simulink model "lab3_ss_nominal_box_sim"  (R2024b)
settings: Solver=ode45  StartTime=0.0  StopTime=20  RelTol=1e-3
undefined symbols (not defined in the file): degs2rpm, deltaSS, DiscIntNeverNeededParam, nominal_K, nominal_Nu, nominal_Nx, rpm2rads, sens, step_amplitude, t0_value, t1_value, Ts, wcSS
libraries: simulink x1
settings Model: Creator=andre  LastModifiedBy=andre

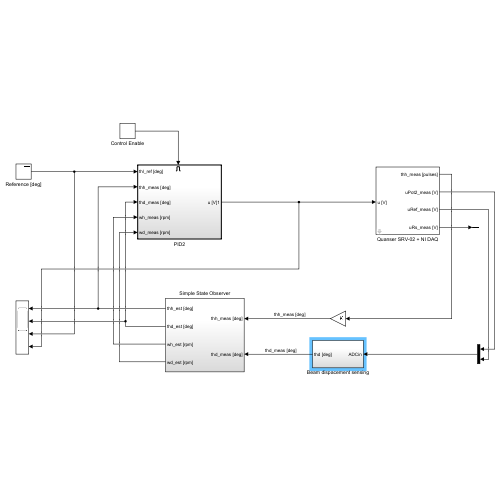
[thumbnail: Simulink's stored preview of the top-level diagram]
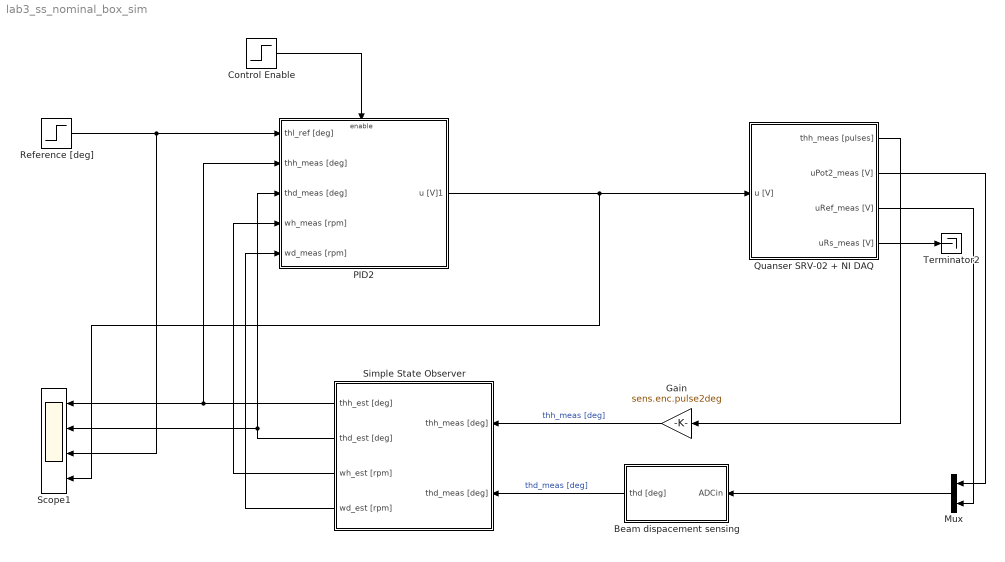
== system lab3_ss_nominal_box_sim ==
  Beam dispacement sensing : Subsystem
  Control Enable : Step  Time=0.7  SampleTime=0
  Gain : Gain  Gain=sens.enc.pulse2deg
  Mux : Mux  Inputs=2
  PID2 : Subsystem
  Quanser SRV-02 + NI DAQ : Subsystem  mask(Quanser SRV-02 (with resonant load) + NI DAQ){Ts=Ts, fricType=Karnopp, lockShaft=off, beamInitPos=10}
      mask prompts: Ts "NI DAQ Sample Time:"; fricType "Friction model"; lockShaft "Lock motor shaft"; beamInitPos "Beam initial position [deg]:"
      mask help: Quanser SRV-02 (with resonant load) + NI DAQ model.
      mask init:
      | %%
      | % Riccardo Antonello (riccardo.antonello@unipd.it)
      | %
      | % April 28, 2020
      | %
      | % Dept. of Information Engineering, University of Padova
      | %
      | 
      | %%  Conversion gains
      | deg2rad = pi/180;                   %   [deg]   -> [rad]
      | rad2deg = 180/pi;                   %   [rad]   -> [deg]
      | 
      | 
      | %%  Sensors data
      | 
      | %   shunt resistor
      | sens.curr.Rs = 0.5;   
      | 
      | %   Hewlett-Packard HEDS-5540#A06 optical encoder
      | sens.enc.ppr = 500*4;                                                   %   pulses per rotation
      | sens.enc.pulse2deg = 360/sens.enc.ppr;                                  %   [pulses] -> [deg]
      | sens.enc.pulse2rad = 2*pi/sens.enc.ppr;                                 %   [pulses] -> [rad]
      | sens.enc.deg2pulse = sens.enc.ppr/360;                                  %   [deg] -> [pulses]
      | sens.enc.rad2pulse = sens.enc.ppr/2/pi;                                 %   [rad] -> [pulses]
      | 
      | %   potentiometer 2 (Spectrol 357-0-0-103) - installed on hub
      | sens.pot2.range.R      = 10e3;                                          %   ohmic value range 
      | sens.pot2.range.V      = 5;                                             %   voltage range
      | sens.pot2.range.th_deg = 340;                                           %   angle range [deg]
      | sens.pot2.range.th     = sens.pot2.range.th_deg * deg2rad;              %   angle range [rad]                           
      | sens.pot2.deg2V        = sens.pot2.range.V / sens.pot2.range.th_deg;    %   sensitivity [V/deg]
      | sens.pot2.rad2V        = sens.pot2.range.V / sens.pot2.range.th;        %   sensitivity [V/rad]
      | sens.pot2.V2deg        = 1/sens.pot2.deg2V;                             %   conversion gain [V] -> [deg]
      | sens.pot2.V2rad        = 1/sens.pot2.rad2V;                             %   conversion gain [V] -> [rad]
      | sens.pot2.noise.var    = 3.5e-7;                                        %   out noise variance [V^2]
      | 
      | 
      | %%  Data acquisition board (daq) data
      | 
      | %   NI PCI-6221 DAC data
      | daq.dac.bits = 16;                                  %   resolution (bits)
      | daq.dac.fs   = 10;                                  %   full scale 
      | daq.dac.q    = 2*daq.dac.fs/(2^daq.dac.bits-1);     %	quantization
      | 
      | %   NI PCI-6221 ADC data
      | daq.adc.bits = 16;                                  %   resolution (bits)
      | daq.adc.fs   = 10;                                  %   full scale (as set in SLDRT Analog Input block)
      | daq.adc.q    = 2*daq.adc.fs/(2^daq.adc.bits-1);     %   quantization   
      | 
      | 
      | %%  Set beam initial position
      | % SRV02Handle = find_system(gcb, ...
      | %     'LookUnderMasks', 'on', ...
      | %     'FindAll', 'on', ...
      | %     'FollowLinks', 'on', ...
      | %     'SearchDepth', '1', ...
      | %     'BlockType', 'ModelReference', ...
      | %     'Name', 'Quanser SRV-02');
      | %
      | % %get_param(SRV02Handle, 'InstanceParameters')
      | % InstanceParams = get_param(SRV02Handle, 'InstanceParameters');
      | % for k = 1:length(InstanceParams)
      | %     if strcmp(InstanceParams(k).Name, 'thb0')
      | %         if lockShaft
      | %             InstanceParams(k).Value = sprintf('%f', beamInitPos);
      | %         else
      | %             InstanceParams(k).Value = sprintf('%f', 0);    
      | %         end
      | %         set_param(SRV02Handle, 'InstanceParameters', InstanceParams);
      | %         break;
      | %     end
      | % end
      | 
      | if lockShaft
      |     thb0 = beamInitPos;
      | else
      |     thb0 = 0;    
      | end
      | 
      | 
      | %%  Mask initialization
      | if lockShaft
      |     
      |     %   find Inport handle
      |     InPortHandle = find_system(gcb, ...
      |         'LookUnderMasks', 'on', ...
      |         'FindAll', 'on', ...
      |         'FollowLinks', 'on', ...
      |         'SearchDepth', '1', ...
      |         'BlockType', 'Inport', ...
      |         'Name', 'u [V]');
      |     
      |     if ~isempty(InPortHandle)
      |     
      |         %   find DAC handle
      |         DACHandle = find_system(gcb, ...
      |             'LookUnderMasks', 'on', ...
      |             'FindAll', 'on', ...
      |             'FollowLinks', 'on', ...
      |             'SearchDepth', '1', ...
      |             'BlockType', 'SubSystem', ...
      |             'Name', 'DAC');  
      | 
      |         %   remove Inport output connection   
      |         InportConn = get_param(InPortHandle, 'PortConnectivity');
      |         delete_line(gcb, InportConn.Position);
      | 
      |         %   remove Inport block
      |         delete_block(InPortHandle);
      | 
      |         %   add Constant block
      |         ConstantHandle = add_block( ...
      |             'simulink/Sources/Constant', [gcb, '/u [V]'], ...
      |             'Position', [20   -37    50   -23], ...
      |             'Value', '0');
      | 
      |         %   connect Constant to DAC block
      |         DACPortHandles = get_param(DACHandle, 'PortHandles');
      |         ConstantPortHandles = get_param(ConstantHandle, 'PortHandles');
      |         add_line(gcb, ConstantPortHandles.Outport(1), DACPortHandles.Inport(1));
      |     
      |     end
      |     
      | else
      |     
      |     %   find Constant handle
      |     ConstantHandle = find_system(gcb, ...
      |         'LookUnderMasks', 'on', ...
      |         'FindAll', 'on', ...
      |         'FollowLinks', 'on', ...
      |         'SearchDepth', '1', ...
      |         'BlockType', 'Constant', ...
      |         'Name', 'u [V]');
      |     
      |     if ~isempty(ConstantHandle)
      |     
      |         %   find DAC handle
      |         DACHandle = find_system(gcb, ...
      |             'LookUnderMasks', 'on', ...
      |             'FindAll', 'on', ...
      |             'FollowLinks', 'on', ...
      |             'SearchDepth', '1', ...
      |             'BlockType', 'SubSystem', ...
      |             'Name', 'DAC');  
      |  
      |         %   remove Constant output connection   
      |         ConstantConn = get_param(ConstantHandle, 'PortConnectivity');
      |         delete_line(gcb, ConstantConn.Position);
      | 
      |         %   remove Inport block
      |         delete_block(ConstantHandle);   
      | 
      |         %   add Inport block
      |         InportHandle = add_block( ...
      |             'simulink/Sources/In1', [gcb, '/u [V]'], ...
      |             'Position', [20   -37    50   -23], ...
      |             'Port', '1');
      | 
      |         %   connect Constant to DAC block
      |         DACPortHandles = get_param(DACHandle, 'PortHandles');
      |         InportPortHandles = get_param(InportHandle, 'PortHandles');
      |         add_line(gcb, InportPortHandles.Outport(1), DACPortHandles.Inport(1));
      |     
      |      end
      |     
      | end
      mask Help:
      | Riccardo Antonello (antonello@dei.unipd.it)
      | 
      | April 28, 2020
      | 
      | Dept. of Information Engineering, University of Padova
      mask TypeOptions fricType: Coulomb + viscous | Karnopp
      mask Callback lockShaft:
      | %   get status of check box
      | lockShaft = get_param(gcb, 'lockShaft');
      | 
      | %   get current value of MaskVisibilities property
      | maskVisibilities = get_param(gcb, 'MaskVisibilities');
      | 
      | %   set visibility of the dialog box element
      | if strcmp(lockShaft, 'on')
      |     maskVisibilities{4} = 'on';
      | else
      |     maskVisibilities{4} = 'off';
      | end
      | 
      | % Set the 'MaskVisibilities' property for each parameter in mask
      | set_param( gcb, 'MaskVisibilities', maskVisibilities);
  Reference [deg] : Step  Time=0  After=step_amplitude  SampleTime=Ts
  Scope1 : Scope  NumInputPorts=4
  Simple State Observer : Subsystem
  Terminator2 : Terminator
  wires:
  Gain/1 -> Simple State Observer/1(thh_meas [deg])  "thh_meas [deg]"
  Reference [deg]/1 -> Scope1/3, PID2/1(thl_ref [deg])
  Quanser SRV-02 + NI DAQ/1(thh_meas [pulses]) -> Gain/1
  Mux/1 -> Beam dispacement sensing/1(ADCin)
  Quanser SRV-02 + NI DAQ/4(uRs_meas [V]) -> Terminator2/1
  Quanser SRV-02 + NI DAQ/3(uRef_meas [V]) -> Mux/2
  Simple State Observer/1(thh_est [deg]) -> PID2/2(thh_meas [deg]), Scope1/1
  Control Enable/1 -> PID2/Enable
  Quanser SRV-02 + NI DAQ/2(uPot2_meas [V]) -> Mux/1
  Beam dispacement sensing/1(thd [deg]) -> Simple State Observer/2(thd_meas [deg])  "thd_meas [deg]"
  PID2/1(u [V]1) -> Quanser SRV-02 + NI DAQ/1(u [V]), Scope1/4
  Simple State Observer/2(thd_est [deg]) -> Scope1/2, PID2/3(thd_meas [deg])
  Simple State Observer/3(wh_est [rpm]) -> PID2/4(wh_meas [rpm])
  Simple State Observer/4(wd_est [rpm]) -> PID2/5(wd_meas [rpm])

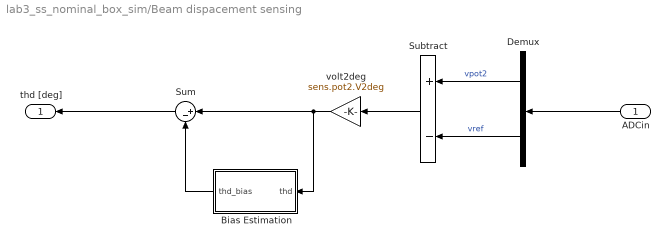
== system lab3_ss_nominal_box_sim/Beam dispacement sensing ==
  ADCin : Inport
  Bias Estimation : Subsystem
  Demux : Demux  Outputs=2
  Subtract : Sum  Inputs=+-
  Sum : Sum  Inputs=|+-
  volt2deg : Gain  Gain=sens.pot2.V2deg
  thd [deg] : Outport
  wires:
  Subtract/1 -> volt2deg/1
  volt2deg/1 -> Sum/1, Bias Estimation/1(thd)
  Sum/1 -> thd [deg]/1
  Bias Estimation/1(thd_bias) -> Sum/2
  ADCin/1 -> Demux/1
  Demux/1 -> Subtract/1  "vpot2"
  Demux/2 -> Subtract/2  "vref"

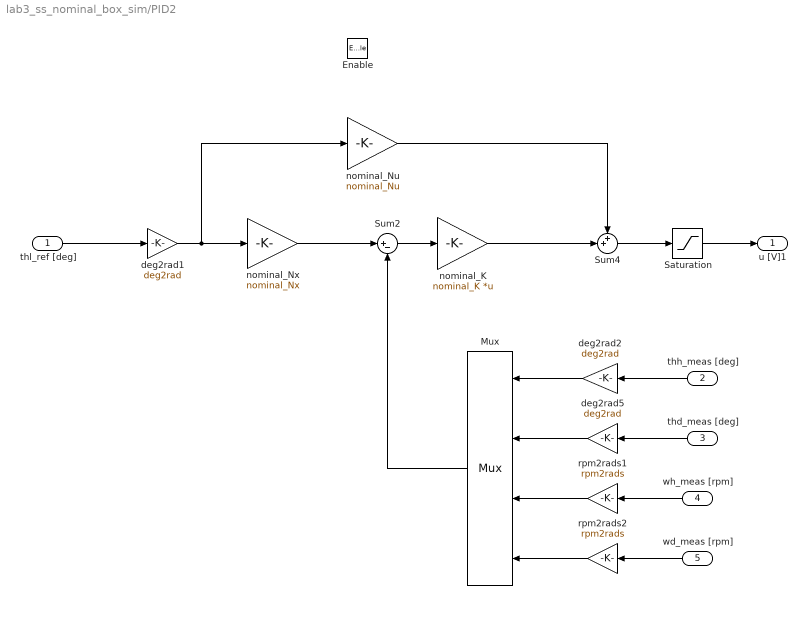
== system lab3_ss_nominal_box_sim/PID2 ==
  thl_ref [deg] : Inport
  thh_meas [deg] : Inport  Port=2
  thd_meas [deg] : Inport  Port=3
  wh_meas [rpm] : Inport  Port=4
  wd_meas [rpm] : Inport  Port=5
  Enable : EnablePort
  Mux : Mux
      settings: DisplayOption=signals
  Saturation : Saturate  UpperLimit=10  LowerLimit=-10
  Sum2 : Sum  Inputs=|+-
  Sum4 : Sum  Inputs=++|
  deg2rad1 : Gain  Gain=deg2rad
  deg2rad2 : Gain  Gain=deg2rad
  deg2rad5 : Gain  Gain=deg2rad
  nominal_K : Gain  Gain=nominal_K  Multiplication=Matrix(K*u)
  nominal_Nu : Gain  Gain=nominal_Nu
  nominal_Nx : Gain  Gain=nominal_Nx
  rpm2rads1 : Gain  Gain=rpm2rads
  rpm2rads2 : Gain  Gain=rpm2rads
  u [V]1 : Outport
  wires:
  wh_meas [rpm]/1 -> rpm2rads1/1
  rpm2rads2/1 -> Mux/4
  nominal_K/1 -> Sum4/2
  rpm2rads1/1 -> Mux/3
  nominal_Nu/1 -> Sum4/1
  deg2rad1/1 -> nominal_Nu/1, nominal_Nx/1
  Saturation/1 -> u [V]1/1
  Sum4/1 -> Saturation/1
  wd_meas [rpm]/1 -> rpm2rads2/1
  thl_ref [deg]/1 -> deg2rad1/1
  thh_meas [deg]/1 -> deg2rad2/1
  thd_meas [deg]/1 -> deg2rad5/1
  nominal_Nx/1 -> Sum2/1
  Mux/1 -> Sum2/2
  Sum2/1 -> nominal_K/1
  deg2rad2/1 -> Mux/1
  deg2rad5/1 -> Mux/2

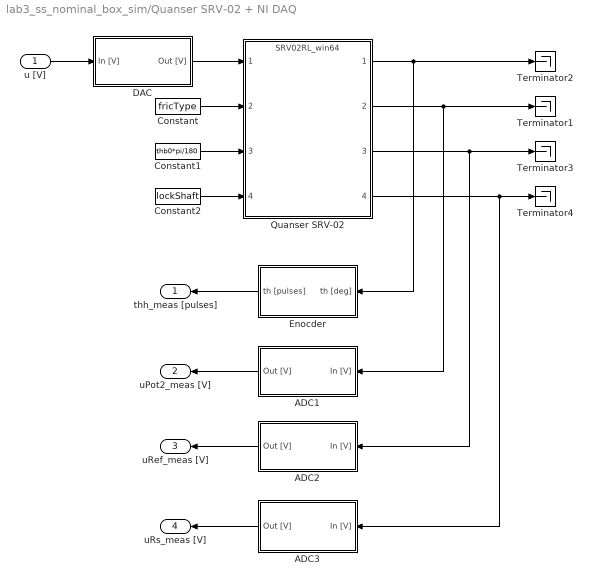
== system lab3_ss_nominal_box_sim/Quanser SRV-02 + NI DAQ ==
  u [V] : Inport
  ADC1 : Subsystem
  ADC2 : Subsystem
  ADC3 : Subsystem
  Constant : Constant  Value=fricType
  Constant1 : Constant  Value=thb0*pi/180  SampleTime=Inf
  Constant2 : Constant  Value=lockShaft  SampleTime=Inf
  DAC : Subsystem
  Enocder : Subsystem
  Quanser SRV-02 : ModelReference  ModelNameDialog=SRV02RL_win64.slxp  ModelReferenceVersion=1.76  CopyOfModelProtected=on
  Terminator{1..4} (4 alike) : Terminator
  thh_meas [pulses] : Outport
  uPot2_meas [V] : Outport  Port=2
  uRef_meas [V] : Outport  Port=3
  uRs_meas [V] : Outport  Port=4
  wires:
  Enocder/1(th [pulses]) -> thh_meas [pulses]/1
  ADC3/1(Out [V]) -> uRs_meas [V]/1
  DAC/1(Out [V]) -> Quanser SRV-02/1
  Quanser SRV-02/2 -> ADC1/1(In [V]), Terminator1/1
  Quanser SRV-02/1 -> Terminator2/1, Enocder/1(th [deg])
  Constant/1 -> Quanser SRV-02/2
  Quanser SRV-02/3 -> ADC2/1(In [V]), Terminator3/1
  ADC1/1(Out [V]) -> uPot2_meas [V]/1
  Constant1/1 -> Quanser SRV-02/3
  Constant2/1 -> Quanser SRV-02/4
  Quanser SRV-02/4 -> ADC3/1(In [V]), Terminator4/1
  ADC2/1(Out [V]) -> uRef_meas [V]/1
  u [V]/1 -> DAC/1(In [V])

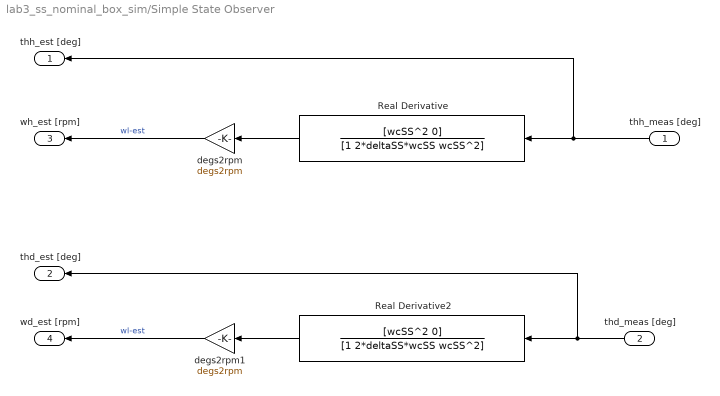
== system lab3_ss_nominal_box_sim/Simple State Observer ==
  thh_meas [deg] : Inport
  thd_meas [deg] : Inport  Port=2
  Real Derivative : TransferFcn  Numerator=[wcSS^2 0]  Denominator=[1 2*deltaSS*wcSS wcSS^2]
  Real Derivative2 : TransferFcn  Numerator=[wcSS^2 0]  Denominator=[1 2*deltaSS*wcSS wcSS^2]
  degs2rpm : Gain  Gain=degs2rpm
  degs2rpm1 : Gain  Gain=degs2rpm
  thh_est [deg] : Outport
  thd_est [deg] : Outport  Port=2
  wh_est [rpm] : Outport  Port=3
  wd_est [rpm] : Outport  Port=4
  wires:
  thd_meas [deg]/1 -> Real Derivative2/1, thd_est [deg]/1
  degs2rpm1/1 -> wd_est [rpm]/1  "wl-est"
  Real Derivative2/1 -> degs2rpm1/1
  degs2rpm/1 -> wh_est [rpm]/1  "wl-est"
  Real Derivative/1 -> degs2rpm/1
  thh_meas [deg]/1 -> thh_est [deg]/1, Real Derivative/1

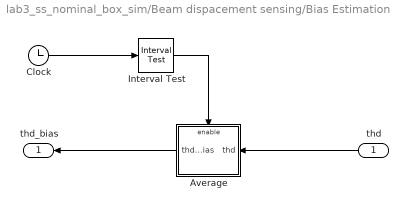
== system lab3_ss_nominal_box_sim/Beam dispacement sensing/Bias Estimation ==
  thd : Inport
  Average : Subsystem
  Clock : Clock
  Interval Test : simulink/Logic and Bit Operations/Interval Test  IntervalClosedRight=on  uplimit=t1_value  IntervalClosedLeft=on  lowlimit=t0_value  OutDataTypeStr=boolean
  thd_bias : Outport
  wires:
  thd/1 -> Average/1(thd)
  Average/1(thd_bias) -> thd_bias/1
  Clock/1 -> Interval Test/1
  Interval Test/1 -> Average/Enable

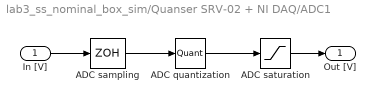
== system lab3_ss_nominal_box_sim/Quanser SRV-02 + NI DAQ/ADC1 ==
  In [V] : Inport
  ADC quantization : Quantizer  QuantizationInterval=daq.adc.q
  ADC sampling : ZeroOrderHold  SampleTime=Ts
  ADC saturation : Saturate  UpperLimit=daq.adc.fs  LowerLimit=-daq.adc.fs
  Out [V] : Outport
  wires:
  ADC saturation/1 -> Out [V]/1
  ADC sampling/1 -> ADC quantization/1
  In [V]/1 -> ADC sampling/1
  ADC quantization/1 -> ADC saturation/1

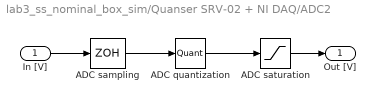
== system lab3_ss_nominal_box_sim/Quanser SRV-02 + NI DAQ/ADC2 ==
  In [V] : Inport
  ADC quantization : Quantizer  QuantizationInterval=daq.adc.q
  ADC sampling : ZeroOrderHold  SampleTime=Ts
  ADC saturation : Saturate  UpperLimit=daq.adc.fs  LowerLimit=-daq.adc.fs
  Out [V] : Outport
  wires:
  ADC quantization/1 -> ADC saturation/1
  In [V]/1 -> ADC sampling/1
  ADC sampling/1 -> ADC quantization/1
  ADC saturation/1 -> Out [V]/1

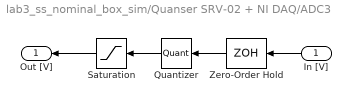
== system lab3_ss_nominal_box_sim/Quanser SRV-02 + NI DAQ/ADC3 ==
  In [V] : Inport
  Quantizer : Quantizer  QuantizationInterval=daq.adc.q
  Saturation : Saturate  UpperLimit=daq.adc.fs  LowerLimit=-daq.adc.fs
  Zero-Order Hold : ZeroOrderHold  SampleTime=Ts
  Out [V] : Outport
  wires:
  Saturation/1 -> Out [V]/1
  In [V]/1 -> Zero-Order Hold/1
  Quantizer/1 -> Saturation/1
  Zero-Order Hold/1 -> Quantizer/1

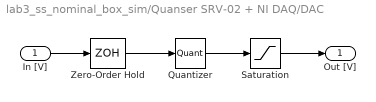
== system lab3_ss_nominal_box_sim/Quanser SRV-02 + NI DAQ/DAC ==
  In [V] : Inport
  Quantizer : Quantizer  QuantizationInterval=daq.dac.q
  Saturation : Saturate  UpperLimit=daq.dac.fs  LowerLimit=-daq.dac.fs
  Zero-Order Hold : ZeroOrderHold  SampleTime=Ts
  Out [V] : Outport
  wires:
  Quantizer/1 -> Saturation/1
  In [V]/1 -> Zero-Order Hold/1
  Zero-Order Hold/1 -> Quantizer/1
  Saturation/1 -> Out [V]/1

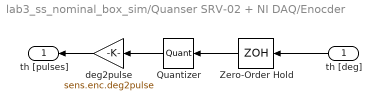
== system lab3_ss_nominal_box_sim/Quanser SRV-02 + NI DAQ/Enocder ==
  th [deg] : Inport
  Quantizer : Quantizer  QuantizationInterval=sens.enc.pulse2deg
  Zero-Order Hold : ZeroOrderHold  SampleTime=Ts
  deg2pulse : Gain  Gain=sens.enc.deg2pulse
  th [pulses] : Outport
  wires:
  Quantizer/1 -> deg2pulse/1
  th [deg]/1 -> Zero-Order Hold/1
  Zero-Order Hold/1 -> Quantizer/1
  deg2pulse/1 -> th [pulses]/1

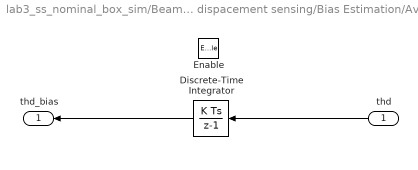
== system lab3_ss_nominal_box_sim/Beam dispacement sensing/Bias Estimation/Average ==
  thd : Inport
  Enable : EnablePort
  Discrete-Time Integrator : DiscreteIntegrator  gainval=1/(t1_value-t0_value)  SampleTime=Ts  ICPrevOutput=DiscIntNeverNeededParam  ICPrevScaledInput=DiscIntNeverNeededParam
  thd_bias : Outport
  wires:
  thd/1 -> Discrete-Time Integrator/1
  Discrete-Time Integrator/1 -> thd_bias/1
